simulink model "cartesianLinearHCW"  (R2023a)
settings: Solver=ode4  StartTime=0.0  StopTime=10.0  FixedStep=dt  RelTol=1e-3
settings Model: Creator=ndelurgio  LastModifiedBy=ndelurgio

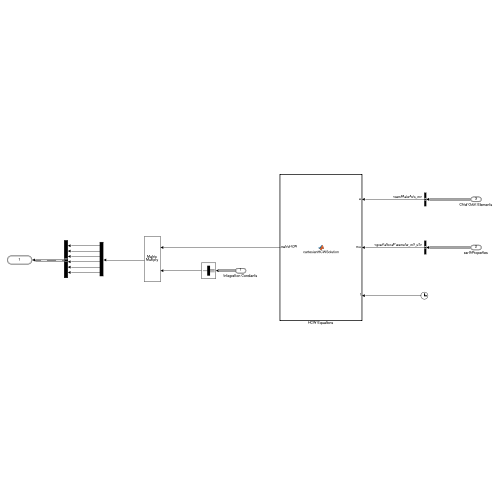
[thumbnail: Simulink's stored preview of the top-level diagram]
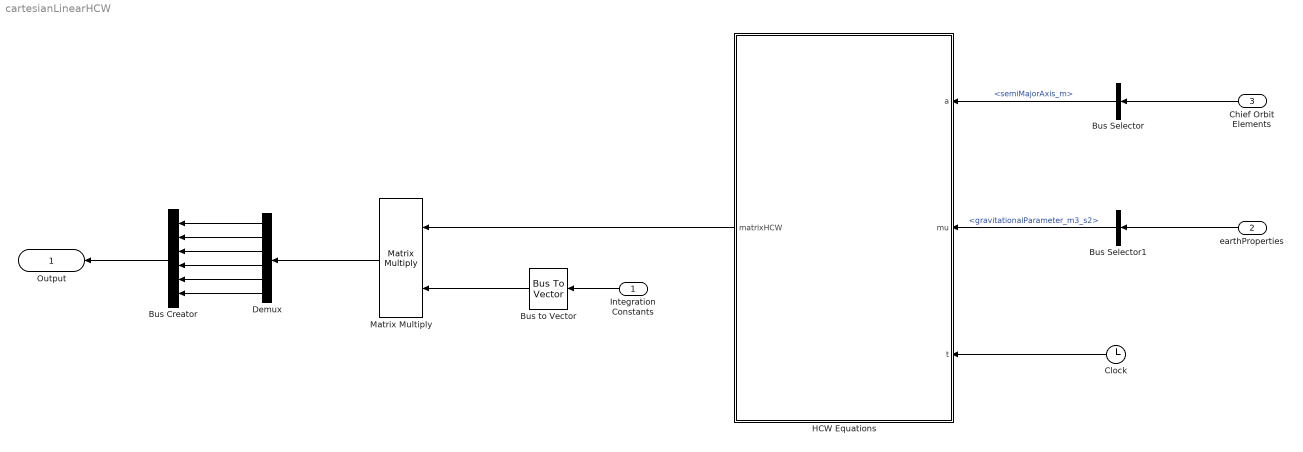
== system cartesianLinearHCW ==
  Integration Constants : Inport  OutDataTypeStr=Bus: integrationConstants_HCW
  earthProperties : Inport  Port=2  OutDataTypeStr=Bus: earthProperties
  Chief Orbit Elements : Inport  Port=3  OutDataTypeStr=Bus: orbitElements
  Bus Creator : BusCreator  Inputs=6  OutDataTypeStr=Bus: relativeCartesianState  NonVirtualBus=on
      settings: InheritFromInputs=off
  Bus Selector : BusSelector  OutputSignals=semiMajorAxis_m
  Bus Selector1 : BusSelector  OutputSignals=gravitationalParameter_m3_s2
  Bus to Vector : BusToVector
  Clock : Clock
  Demux : Demux  Outputs=6
  HCW Equations : MATLAB Function  TreatAsAtomicUnit=on
  Matrix Multiply : Product  Multiplication=Matrix(*)
  Output : Outport  OutDataTypeStr=Bus: relativeCartesianState
  wires:
  Integration Constants/1 -> Bus to Vector/1
  Chief Orbit Elements/1 -> Bus Selector/1
  Bus Selector/1 -> HCW Equations/1(a)  "<semiMajorAxis_m>"
  earthProperties/1 -> Bus Selector1/1
  Bus Selector1/1 -> HCW Equations/2(mu)  "<gravitationalParameter_m3_s2>"
  Clock/1 -> HCW Equations/3(t)
  HCW Equations/1(matrixHCW) -> Matrix Multiply/1
  Demux/1 -> Bus Creator/1
  Demux/2 -> Bus Creator/2
  Demux/3 -> Bus Creator/3
  Demux/4 -> Bus Creator/4
  Demux/5 -> Bus Creator/5
  Demux/6 -> Bus Creator/6
  Bus Creator/1 -> Output/1
  Matrix Multiply/1 -> Demux/1
  Bus to Vector/1 -> Matrix Multiply/2

== matlab function cartesianLinearHCW/HCW Equations ==
  data: matrixHCW output; a input; mu input; t input
function matrixHCW = cartesianHCWSolution(a, mu, t)

matrixHCW = cartesianHCWSolution(a, mu, t);

end
